simulink model "On_off_control"  (Simulink 9.3)
settings: Solver=VariableStepAuto  StartTime=0.0  StopTime=500  RelTol=1e-3  EnableMultiTasking=on
StartFcn:
  | clear all
libraries: realtime_pacer_lib x1
settings Model: Creator=johnh  LastModifiedBy=hgarnier
settings DataIOCC: SaveFormat=Dataset  SignalLoggingSaveFormat=Dataset
settings DebuggingCC: UnderspecifiedInitializationDetection=Simplified  MergeDetectMultiDrivingBlocksExec=error  FcnCallInpInsideContextMsg=error  PregeneratedLibrarySubsystemCodeDiagnostic=none
settings HardwareCC: ProdBitPerPointer=64  ProdBitPerSizeT=64  ProdBitPerPtrDiffT=64  ProdLargestAtomicFloat=Float  ProdIntDivRoundTo=Zero  ProdEndianess=LittleEndian  ProdWordSize=64  ProdHWDeviceType=Intel->x86-64 (Windows64)
settings ModelReferenceCC: PropagateSignalLabelsOutOfModel=on
settings GRTTargetCC: GeneratePreprocessorConditionals=Disable all  CombineOutputUpdateFcns=on  GRTInterface=off

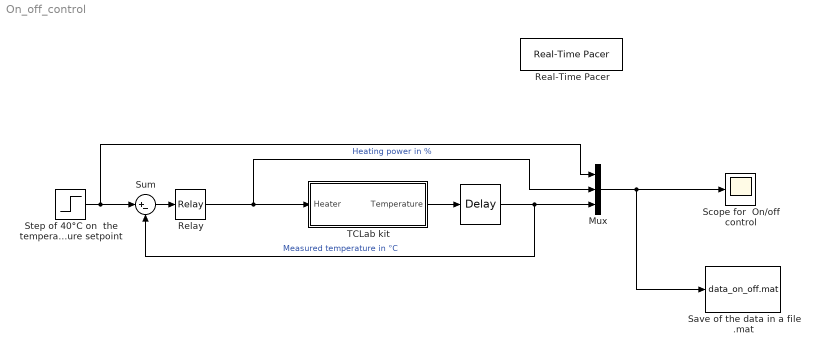
== system On_off_control ==
  " " : TransportDelay
  Mux : Mux  Inputs=3
  Real-Time Pacer : realtime_pacer_lib/Real-Time Pacer  simTimePerRealTime=1
  Relay : Relay  OffSwitchValue=-eps  OnOutputValue=100
  Save of the data in a file .mat : ToFile  Filename=data_on_off.mat  MatrixName=data_on_off
  Scope for  On/off control : Scope
  Step of 40°C on  the temperature setpoint : Step  Time=25  After=40  SampleTime=0
  Sum : Sum  Inputs=|+-
  "TCLab kit " : Subsystem
  wires:
  Relay/1 -> "TCLab kit "/1(Heater), Mux/2  "Heating power in %"
  Mux/1 -> Save of the data in a file .mat/1, Scope for  On/off control/1
  Sum/1 -> Relay/1
  Step of 40°C on  the temperature setpoint/1 -> Mux/1, Sum/1
  "TCLab kit "/1(Temperature) -> " "/1
  " "/1 -> Mux/3, Sum/2  "Measured temperature in °C"

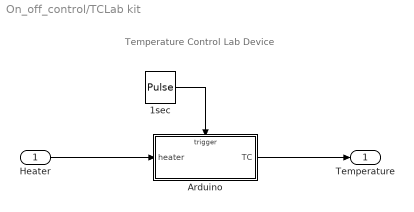
== system On_off_control/TCLab kit  ==
  note: Temperature Control Lab Device
  Heater : Inport
  1sec : DiscretePulseGenerator  PulseType=Time based  Period=1  PulseWidth=50
  Arduino : Subsystem  TreatAsAtomicUnit=on
  Temperature : Outport
  wires:
  1sec/1 -> Arduino/Trigger
  Arduino/1(TC) -> Temperature/1
  Heater/1 -> Arduino/1(heater)

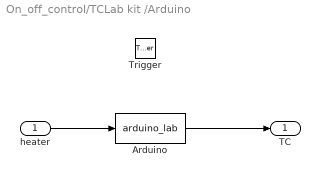
== system On_off_control/TCLab kit /Arduino ==
  heater : Inport
  Trigger : TriggerPort  VariantControl=Variant
  Arduino : MATLABFcn  MATLABFcn=arduino_lab
  TC : Outport  InitialOutput=23
  wires:
  heater/1 -> Arduino/1
  Arduino/1 -> TC/1
